simulink model "LQR"  (R2021b)
settings: Solver=VariableStepAuto  StartTime=0.0  StopTime=tsim  RelTol=1e-3
values from neighbouring files (symbols this model uses):
  A = [   -1/Ti(1),   0,          Ai(1)/(Ai(3)*Ti(3)),    0;          0,          -1/Ti(2),   0,                      Ai(2)/(Ai(3)*Ti(3));          0,          0,          -1/Ti(3),               0;          0,          0,          0,                      -1/Ti(4)]    [fcn_matlab.m]
  B = [gamma(1)*k(1)/Ai(1),       0;      0,                          gamma(2)*k(2)/Ai(2);      0,                          (1-gamma(2))*k(2)/Ai(3);      (1-gamma(1))*k(1)/Ai(4),    0]    [fcn_matlab.m]
  C = [kc,  0,      0, 0;       0,     kc,   0, 0]    [fcn_matlab.m]
  ref = [0,0,0,0]    [fcn_matlab.m]
  x0 = [40, 40, 40, 40]    [fcn_matlab.m]
undefined symbols (not defined in the file or in its folder): K
settings Model: Creator=nkantorn  LastModifiedBy=joaqu
settings DebuggingCC: UnconnectedInputMsg=none  UnconnectedOutputMsg=none  UnconnectedLineMsg=none
settings ModelReferenceCC: EnableRefExpFcnMdlSchedulingChecks=off
settings RTWCC: DLArmComputeVersion=20.02.1

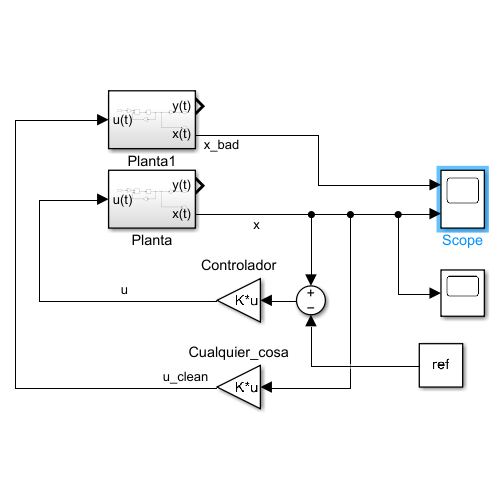
[thumbnail: Simulink's stored preview of the top-level diagram]
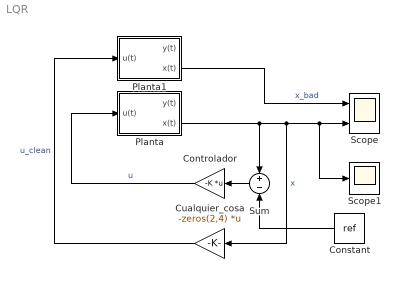
== system LQR ==
  Constant : Constant  Value=ref
  Controlador : Gain  Gain=-K  Multiplication=Matrix(K*u)
  Cualquier_cosa : Gain  Gain=-zeros(2,4)  Multiplication=Matrix(K*u)
  Planta : Subsystem
  Planta1 : Subsystem
  Scope : Scope  NumInputPorts=2
  Scope1 : Scope
  Sum : Sum  Inputs=+|-
  wires:
  Planta/2(x(t)) -> Sum/1, Cualquier_cosa/1, Scope1/1, Scope/2  "x"
  Controlador/1 -> Planta/1(u(t))  "u"
  Cualquier_cosa/1 -> Planta1/1(u(t))  "u_clean"
  Planta1/2(x(t)) -> Scope/1  "x_bad"
  Sum/1 -> Controlador/1
  Constant/1 -> Sum/2

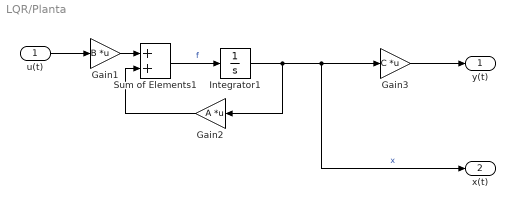
== system LQR/Planta ==
  u(t) : Inport
  Gain1 : Gain  Gain=B  Multiplication=Matrix(K*u)
  Gain2 : Gain  Gain=A  Multiplication=Matrix(K*u)
  Gain3 : Gain  Gain=C  Multiplication=Matrix(K*u)
  Integrator1 : Integrator  InitialCondition=x0
  Sum of Elements1 : Sum
  y(t) : Outport
  x(t) : Outport  Port=2
  wires:
  Gain3/1 -> y(t)/1
  u(t)/1 -> Gain1/1
  Sum of Elements1/1 -> Integrator1/1  "f"
  Integrator1/1 -> Gain3/1, x(t)/1, Gain2/1  "x"
  Gain1/1 -> Sum of Elements1/1
  Gain2/1 -> Sum of Elements1/2

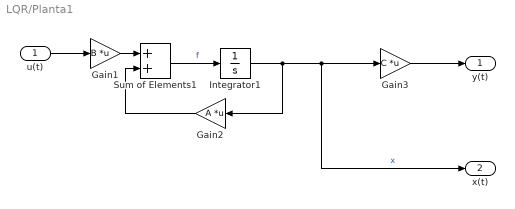
== system LQR/Planta1 ==
  u(t) : Inport
  Gain1 : Gain  Gain=B  Multiplication=Matrix(K*u)
  Gain2 : Gain  Gain=A  Multiplication=Matrix(K*u)
  Gain3 : Gain  Gain=C  Multiplication=Matrix(K*u)
  Integrator1 : Integrator  InitialCondition=x0
  Sum of Elements1 : Sum
  y(t) : Outport
  x(t) : Outport  Port=2
  wires:
  Gain3/1 -> y(t)/1
  u(t)/1 -> Gain1/1
  Sum of Elements1/1 -> Integrator1/1  "f"
  Integrator1/1 -> Gain3/1, x(t)/1, Gain2/1  "x"
  Gain1/1 -> Sum of Elements1/1
  Gain2/1 -> Sum of Elements1/2
